simulink model "MCU_vectorControl_dsPIC33CK256MP508_LVMC"  (R2024a)
settings: Solver=FixedStepDiscrete  StartTime=0.0  StopTime=10.0  FixedStep=50e-6  RelTol=1e-3  EnableMultiTasking=on
undefined symbols (not defined in the file or in its folder): A0, A4, AN0, AN1, B0, B2, Bias1, Bias2, C12, C13, C14, C7, control, D11, D12, D13, D14, D5, D6, D7, diff, DiscIntNeverNeededParam, inverter, Max, MaxPer, model, ms, NumBits1, NumBits2, P20, P32, P55, P60, P61, P62, P69, P70, P71, P75, P76, P77, P78, Pin, pmsm, PosRange1, PosRange2, PWM1max, Resol, s, Slope1, Slope2, us
libraries: simulink x54, MCHP_Blockset x25
(part 3 of 4)

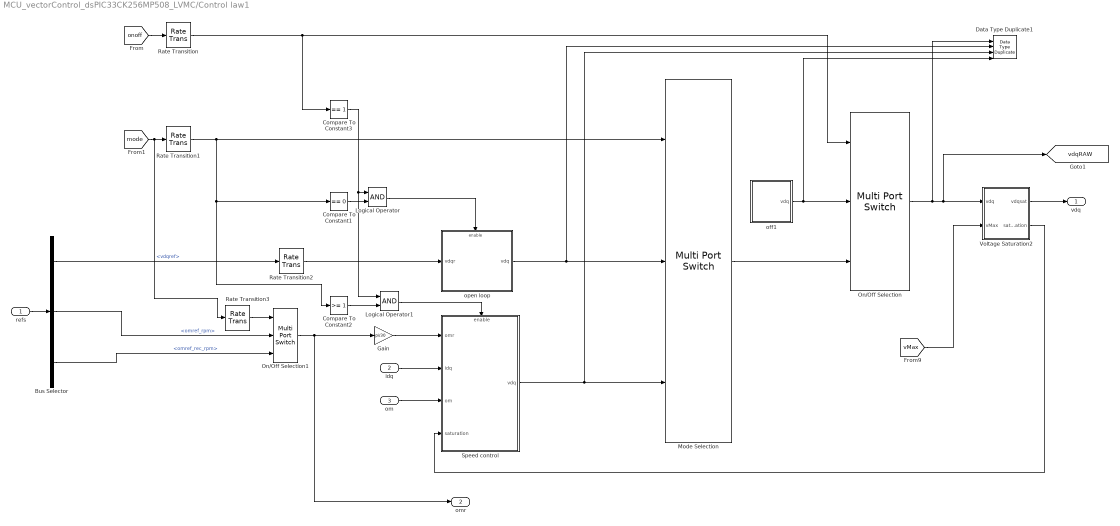
== system MCU_vectorControl_dsPIC33CK256MP508_LVMC/Control law1 ==
  refs : Inport
  idq : Inport  Port=2
  om : Inport  Port=3
  Bus Selector : BusSelector  OutputSignals=vdqref,omref.omref_rpm,omref.omref_rec_rpm
  Compare To Constant1 : simulink/Logic and Bit Operations/Compare To Constant  relop===  const=0  OutDataTypeStr=boolean
  Compare To Constant2 : simulink/Logic and Bit Operations/Compare To Constant  relop=>=  const=1  OutDataTypeStr=boolean
  Compare To Constant3 : simulink/Logic and Bit Operations/Compare To Constant  relop===  const=1  OutDataTypeStr=boolean
  Data Type Duplicate1 : DataTypeDuplicate  NumInputPorts=5
  Gain : Gain  Gain=pi/30  OutDataTypeStr=Inherit: Inherit via back propagation
  Logical Operator : Logic  AllPortsSameDT=off  OutDataTypeStr=boolean
  Logical Operator1 : Logic  AllPortsSameDT=off  OutDataTypeStr=boolean
  Mode Selection : MultiPortSwitch  DataPortOrder=Zero-based contiguous  Inputs=2  DiagnosticForDefault=None  zeroidx=on  SaturateOnIntegerOverflow=off  InputSameDT=off
  On/Off Selection : MultiPortSwitch  DataPortOrder=Zero-based contiguous  Inputs=2  DiagnosticForDefault=None  zeroidx=on  SaturateOnIntegerOverflow=off  InputSameDT=off
  On/Off Selection1 : MultiPortSwitch  DataPortOrder=Specify indices  Inputs=2  DataPortIndices={1,2}  DiagnosticForDefault=None  SaturateOnIntegerOverflow=off  InputSameDT=off
  Rate Transition{,1..3} (4 alike) : RateTransition
  Speed control : Subsystem
      settings: LibrarySourceBlock=insa_control_base/Current Control  PortSchema="{\"entries\":[{\"content\":{\"sides\":[{\"content\":{\"connectorIds\":[\"In1\",\"In2\",\"In3\",\"In4\"]},\"type\":\"ConnectorPlacement.EquallySpacedRectSide\",\"uuid\":\"e7aaa2d5-acdd-4a4d-91b1-423dc6f26e4f\"},{\"content\":{\"connectorIds\":[\"Out1\"],\"side\":\"RIGHT\"},\"type\":\"ConnectorPlacement.EquallySpacedRectSide\",\"uuid\":\"81691e4d-c138-404c-a913-2433211e99ad\"},{\"content\":{\"connectorIds\":[\"In5\"],\"side\":\"TOP\"},\"type\":\"ConnectorPlacement.EquallySpacedRectSide\",\"uuid\":\"67eaf657-96ad-4741-9677-f3dc17f9f096\"}]},\"type\":\"ConnectorPlacement.EquallySpacedConnector\",\"uuid\":\"09d68ba6-6bd5-4801-b033-56cd43b3cecf\"}],\"packageUris\":[\"http://schema.mathworks.com/mf0/Connector/R2020b\"],\"version\":\"1.0\"}"
  Voltage Saturation2 : Subsystem
  off1 : Subsystem
  open loop : Subsystem
  vdq : Outport  VectorParamsAs1DForOutWhenUnconnected=off
  omr : Outport  Port=2
  tag scope: vdqRAW=global
  wires:
  Bus Selector/1 -> Rate Transition2/1  "<vdqref>"
  [mode] -> Rate Transition1/1, Rate Transition3/1
  refs/1 -> Bus Selector/1
  Bus Selector/2 -> On/Off Selection1/2  "<omref_rpm>"
  Bus Selector/3 -> On/Off Selection1/3  "<omref_rec_rpm>"
  On/Off Selection1/1 -> omr/1, Gain/1
  Rate Transition3/1 -> On/Off Selection1/1
  [vMax] -> Voltage Saturation2/2(vMax)
  On/Off Selection/1 -> Voltage Saturation2/1(vdq), [vdqRAW], Data Type Duplicate1/2
  Speed control/1(vdq) -> Mode Selection/3, Data Type Duplicate1/4
  Voltage Saturation2/2(saturation) -> Speed control/4(saturation)
  idq/1 -> Speed control/2(idq)
  om/1 -> Speed control/3(om)
  Logical Operator1/1 -> Speed control/5(enable)
  Compare To Constant3/1 -> Logical Operator/1, Logical Operator1/1
  Compare To Constant1/1 -> Logical Operator/2
  [onoff] -> Rate Transition/1
  open loop/1(vdq) -> Mode Selection/2, Data Type Duplicate1/3
  off1/1(vdq) -> On/Off Selection/2, Data Type Duplicate1/5
  Mode Selection/1 -> On/Off Selection/3
  Logical Operator/1 -> open loop/Enable
  Compare To Constant2/1 -> Logical Operator1/2
  Voltage Saturation2/1(vdqsat) -> vdq/1
  Rate Transition/1 -> Compare To Constant3/1, On/Off Selection/1
  Rate Transition1/1 -> Mode Selection/1, Compare To Constant2/1, Compare To Constant1/1
  Rate Transition2/1 -> open loop/1(vdqr)
  Gain/1 -> Speed control/1(omr)

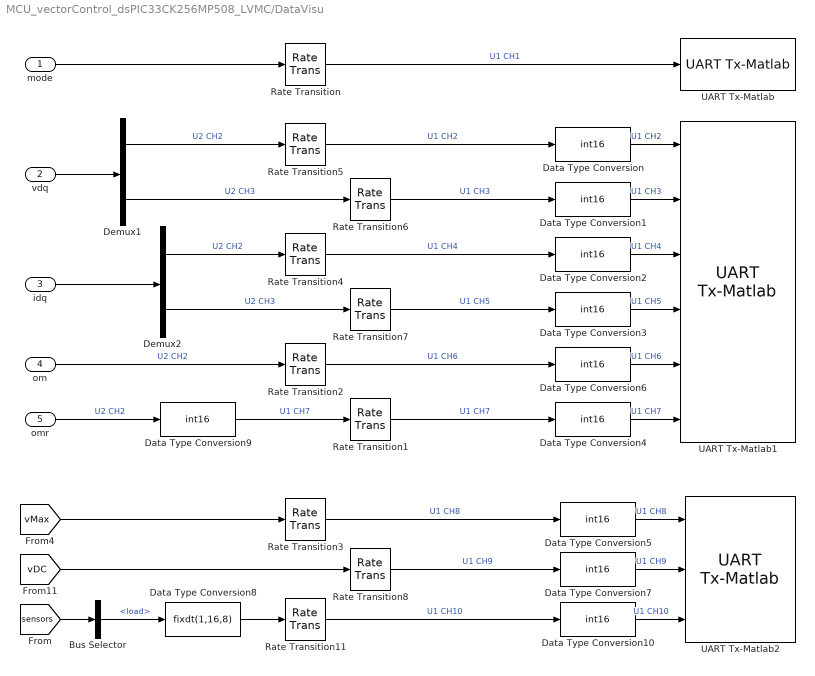
== system MCU_vectorControl_dsPIC33CK256MP508_LVMC/DataVisu ==
  mode : Inport
  vdq : Inport  Port=2
  idq : Inport  Port=3
  om : Inport  Port=4
  omr : Inport  Port=5
  Bus Selector : BusSelector  OutputSignals=MCU.load
  Data Type Conversion{,1..7,10} (9 alike) : DataTypeConversion  OutDataTypeStr=int16  ConvertRealWorld=Stored Integer (SI)  SaturateOnIntegerOverflow=off  RndMeth=Floor
  Data Type Conversion8 : DataTypeConversion  OutDataTypeStr=fixdt(1,16,8)  SaturateOnIntegerOverflow=off  RndMeth=Floor
  Data Type Conversion9 : DataTypeConversion  OutDataTypeStr=int16  SaturateOnIntegerOverflow=off  RndMeth=Floor
  Demux1 : Demux  Outputs=2
  Demux2 : Demux  Outputs=2
  Rate Transition{,1..8,11} (10 alike) : RateTransition
  UART Tx-Matlab : MCHP_Blockset/BUS UART/UART Tx-Matlab  UART_REF=1  CHANNELS=[1]  AllOrNothing=off  SampleTime=.01  MCHP_MASTERLINK=MCU_vectorControl_dsPIC33CK256MP508_LVMC/BOARD dsPIC33CK LVMC/Microchip Master  MCHP_COMPILED_INFO="CompiledSampleTime= [0.010000000000000000208   0 ];CompiledInportDataTypes=[  3 ];CompiledInportDataWidth=[1];"
      settings: SourceProductName=MPLAB Device Blocks for Simulink
  UART Tx-Matlab1 : MCHP_Blockset/BUS UART/UART Tx-Matlab  UART_REF=1  CHANNELS=[2:7]  AllOrNothing=off  SampleTime=0.001  MCHP_MASTERLINK=MCU_vectorControl_dsPIC33CK256MP508_LVMC/BOARD dsPIC33CK LVMC/Microchip Master  MCHP_COMPILED_INFO="CompiledSampleTime= [0.0010000000000000000208   0 ];CompiledInportDataTypes=[  4   4   4   4   4   4 ];CompiledInportDataWidth=[1  1  1  1  1  1];"
      settings: SourceProductName=MPLAB Device Blocks for Simulink
  UART Tx-Matlab2 : MCHP_Blockset/BUS UART/UART Tx-Matlab  UART_REF=1  CHANNELS=[8:10]  AllOrNothing=off  SampleTime=.01  MCHP_MASTERLINK=MCU_vectorControl_dsPIC33CK256MP508_LVMC/BOARD dsPIC33CK LVMC/Microchip Master  MCHP_COMPILED_INFO="CompiledSampleTime= [0.010000000000000000208   0 ];CompiledInportDataTypes=[  4   4   4 ];CompiledInportDataWidth=[1  1  1];"
      settings: SourceProductName=MPLAB Device Blocks for Simulink
  wires:
  vdq/1 -> Demux1/1
  idq/1 -> Demux2/1
  Demux2/2 -> Rate Transition7/1  "U2 CH3"
  Demux2/1 -> Rate Transition4/1  "U2 CH2"
  Rate Transition5/1 -> Data Type Conversion/1  "U1 CH2"
  Demux1/2 -> Rate Transition6/1  "U2 CH3"
  Rate Transition6/1 -> Data Type Conversion1/1  "U1 CH3"
  Rate Transition4/1 -> Data Type Conversion2/1  "U1 CH4"
  Demux1/1 -> Rate Transition5/1  "U2 CH2"
  Rate Transition7/1 -> Data Type Conversion3/1  "U1 CH5"
  Rate Transition2/1 -> Data Type Conversion6/1  "U1 CH6"
  om/1 -> Rate Transition2/1  "U2 CH2"
  Rate Transition/1 -> UART Tx-Matlab/1  "U1 CH1"
  mode/1 -> Rate Transition/1
  omr/1 -> Data Type Conversion9/1  "U2 CH2"
  Rate Transition1/1 -> Data Type Conversion4/1  "U1 CH7"
  [vDC] -> Rate Transition8/1
  [vMax] -> Rate Transition3/1
  Rate Transition3/1 -> Data Type Conversion5/1  "U1 CH8"
  Rate Transition8/1 -> Data Type Conversion7/1  "U1 CH9"
  Bus Selector/1 -> Data Type Conversion8/1  "<load>"
  Rate Transition11/1 -> Data Type Conversion10/1  "U1 CH10"
  [sensors] -> Bus Selector/1
  Data Type Conversion8/1 -> Rate Transition11/1
  Data Type Conversion3/1 -> UART Tx-Matlab1/4  "U1 CH5"
  Data Type Conversion2/1 -> UART Tx-Matlab1/3  "U1 CH4"
  Data Type Conversion6/1 -> UART Tx-Matlab1/5  "U1 CH6"
  Data Type Conversion4/1 -> UART Tx-Matlab1/6  "U1 CH7"
  Data Type Conversion/1 -> UART Tx-Matlab1/1  "U1 CH2"
  Data Type Conversion1/1 -> UART Tx-Matlab1/2  "U1 CH3"
  Data Type Conversion5/1 -> UART Tx-Matlab2/1  "U1 CH8"
  Data Type Conversion10/1 -> UART Tx-Matlab2/3  "U1 CH10"
  Data Type Conversion7/1 -> UART Tx-Matlab2/2  "U1 CH9"
  Data Type Conversion9/1 -> Rate Transition1/1  "U1 CH7"

== system MCU_vectorControl_dsPIC33CK256MP508_LVMC/Heart-beat 5Hz Blinking ==
  Delay : Delay  DelayLength=1  InitialCondition=0  SampleTime=.1
  Logical Operator : Logic  Operator=NOT  AllPortsSameDT=off  OutDataTypeStr=boolean
  Rate Transition2 : RateTransition  Deterministic=off  OutPortSampleTime=0.01
  LED1 : Outport  VectorParamsAs1DForOutWhenUnconnected=off
  wires:
  Delay/1 -> Logical Operator/1
  Logical Operator/1 -> Delay/1, Rate Transition2/1
  Rate Transition2/1 -> LED1/1

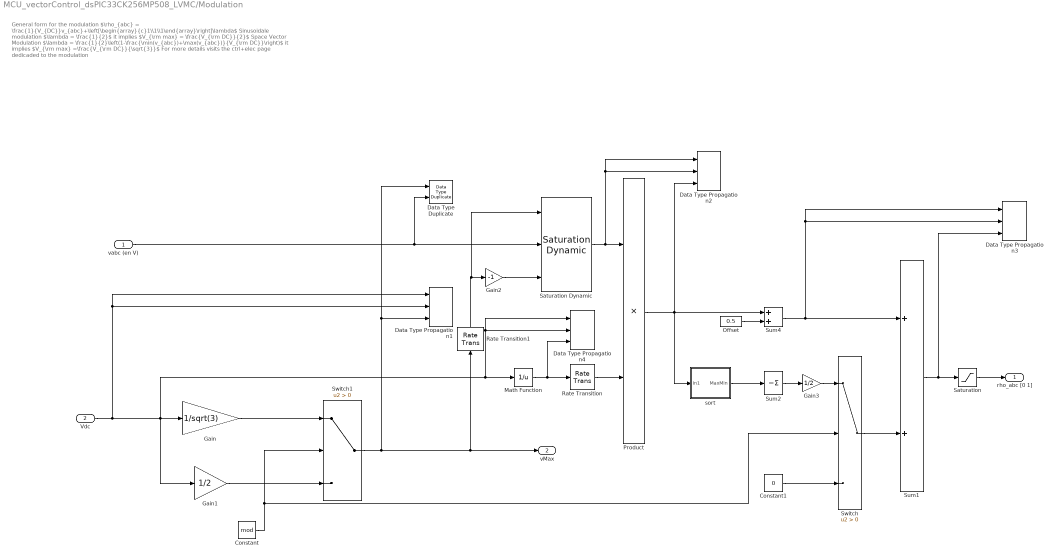
== system MCU_vectorControl_dsPIC33CK256MP508_LVMC/Modulation ==
  note: General form for the modulation
      | $\rho_{abc} = \frac{1}{V_{DC}}v_{abc}+\left[\begin{array}{c}1\\1\\1\end{array}\right]\lambda$
      | Sinusoidale modulation
      | $\lambda = \frac{1}{2}$ it implies $V_{\rm max} = \frac{V_{\rm DC}}{2}$
      | Space Vector Modulation
      | $\lambda = \frac{1}{2}\left(1-\frac{\min(v_{abc})+\max(v_{abc})}{V_{\rm DC}}\right)$ it implies $V_{\rm max} =\frac{V_{\rm DC}}{\sqrt{3}}$
      | For more details visits the ctrl+elec page dedicaded to the modulation
  "vabc (en V) " : Inport
  Vdc : Inport  Port=2
  Constant : Constant  Value=mod  OutDataTypeStr=boolean
  Constant1 : Constant  Value=0  OutDataTypeStr=Inherit: Inherit via back propagation
  Data Type Duplicate : DataTypeDuplicate
  Data Type Propagation1 : simulink/Signal Attributes/Data Type Propagation  PropDataType=fixdt(1, 16)  IfRefDouble=double  IfRefSingle=single  IsSigned=TRUE  NumBitsBase=max([NumBits1 NumBits2])  NumBitsMult=1  NumBitsAdd=0  NumBitsAllowFinal=[1:128]  PropScaling=2^-(15-ceil(log2(inverter.vDC/sqrt(3))))  ValuesUsedBestPrec=[100 -100]  SlopeBase=max([PosRange1 PosRange2])  SlopeMult=1/sqrt(3)  SlopeAdd=0  BiasBase=Bias1  BiasMult=1  BiasAdd=0
  Data Type Propagation2 : simulink/Signal Attributes/Data Type Propagation  PropDataType=fixdt(1, 16)  IfRefDouble=double  IfRefSingle=single  IsSigned=TRUE  NumBitsBase=max([NumBits1 NumBits2])  NumBitsMult=1  NumBitsAdd=0  NumBitsAllowFinal=[1:128]  PropScalingMode=Specify via dialog  PropScaling=2^-14  ValuesUsedBestPrec=[100 -100]  SlopeBase=Slope1/Slope2  SlopeMult=1  SlopeAdd=0  BiasBase=Bias1  BiasMult=1  BiasAdd=0
  Data Type Propagation3 : simulink/Signal Attributes/Data Type Propagation  PropDataType=fixdt(1, 16)  IfRefDouble=double  IfRefSingle=single  IsSigned=FALSE  NumBitsBase=max([NumBits1 NumBits2])  NumBitsMult=1  NumBitsAdd=0  NumBitsAllowFinal=[1:128]  PropScalingMode=Specify via dialog  PropScaling=2^-14  ValuesUsedBestPrec=[100 -100]  SlopeBase=Slope1/Slope2  SlopeMult=1  SlopeAdd=0  BiasBase=Bias1  BiasMult=1  BiasAdd=0
  Data Type Propagation4 : simulink/Signal Attributes/Data Type Propagation  PropDataType=fixdt(1, 16)  IfRefDouble=double  IfRefSingle=single  IsSigned=FALSE  NumBitsBase=max([NumBits1 NumBits2])  NumBitsMult=1  NumBitsAdd=0  NumBitsAllowFinal=[1:128]  PropScalingMode=Specify via dialog  PropScaling=2^-16  ValuesUsedBestPrec=[100 -100]  SlopeBase=max([PosRange1 PosRange2])  SlopeMult=1/sqrt(3)  SlopeAdd=0  BiasBase=Bias1  BiasMult=1  BiasAdd=0
  Gain : Gain  Gain=1/sqrt(3)  OutDataTypeStr=Inherit: Same as input
  Gain1 : Gain  Gain=1/2  OutDataTypeStr=Inherit: Same as input
  Gain2 : Gain  Gain=-1  ParamDataTypeStr=int16  OutDataTypeStr=Inherit: Inherit via back propagation
  Gain3 : Gain  Gain=1/2  OutDataTypeStr=Inherit: Same as input
  Math Function : Math  Operator=reciprocal  OutputSignalType=real  OutDataTypeStr=Inherit: Inherit via back propagation  SaturateOnIntegerOverflow=off
  "Offset " : Constant  Value=0.5  OutMin=[0]  OutMax=[1]  OutDataTypeStr=Inherit: Inherit via back propagation
  Product : Product  Inputs=**  OutDataTypeStr=Inherit: Inherit via back propagation  SaturateOnIntegerOverflow=on
  Rate Transition : RateTransition
  Rate Transition1 : RateTransition
  Saturation : Saturate  UpperLimit=1  LowerLimit=0
  Saturation Dynamic : simulink/Discontinuities/Saturation Dynamic  OutMin=[]  OutMax=[]  OutDataTypeStr=Inherit: Same as second input  OutDataType=fixdt(1, 16)  OutScaling=2^-10  DoSatur=off
  Sum1 : Sum  OutMin=[0]  OutMax=[1]  OutDataTypeStr=Inherit: Inherit via back propagation  InputSameDT=on  SaturateOnIntegerOverflow=on
  Sum2 : Sum  Inputs=-  OutMin=[-1]  OutMax=[1]  InputSameDT=on  SaturateOnIntegerOverflow=on  OutDataTypeStr=Inherit: Same as first input
  Sum4 : Sum  OutMin=[-1]  OutMax=[1]  InputSameDT=on  SaturateOnIntegerOverflow=on  OutDataTypeStr=Inherit: Same as first input
  Switch : Switch  Criteria=u2 > Threshold  SaturateOnIntegerOverflow=off  InputSameDT=off
  Switch1 : Switch  Criteria=u2 > Threshold  OutDataTypeStr=Inherit: Inherit via back propagation  SaturateOnIntegerOverflow=off  InputSameDT=off
  sort : Subsystem
  rho_abc [0 1] : Outport  VectorParamsAs1DForOutWhenUnconnected=off
  vMax : Outport  Port=2  VectorParamsAs1DForOutWhenUnconnected=off
  wires:
  Sum1/1 -> Saturation/1, Data Type Propagation3/3
  Vdc/1 -> Data Type Propagation1/2, Data Type Propagation1/1, Gain/1, Math Function/1, Data Type Propagation4/2, Data Type Propagation4/1, Gain1/1
  Gain3/1 -> Switch/1
  Saturation/1 -> rho_abc [0 1]/1
  Saturation Dynamic/1 -> Product/1, Data Type Propagation2/1, Data Type Propagation2/2
  Gain1/1 -> Switch1/3
  Gain/1 -> Switch1/1
  sort/1(MaxMin) -> Sum2/1
  Sum2/1 -> Gain3/1
  Sum4/1 -> Data Type Propagation3/2, Data Type Propagation3/1, Sum1/1
  Constant1/1 -> Switch/3
  Switch/1 -> Sum1/2
  "Offset "/1 -> Sum4/2
  Product/1 -> Data Type Propagation2/3, Sum4/1, sort/1(In1)
  Gain2/1 -> Saturation Dynamic/3
  Math Function/1 -> Data Type Propagation4/3, Rate Transition/1
  Switch1/1 -> Rate Transition1/1, vMax/1, Data Type Propagation1/3, Data Type Duplicate/1
  Constant/1 -> Switch1/2, Switch/2
  "vabc (en V) "/1 -> Data Type Duplicate/2, Saturation Dynamic/2
  Rate Transition/1 -> Product/2
  Rate Transition1/1 -> Saturation Dynamic/1, Gain2/1

== system MCU_vectorControl_dsPIC33CK256MP508_LVMC/Motor Choice + Gain Tunning ==

== system MCU_vectorControl_dsPIC33CK256MP508_LVMC/Park ==
  xab(c) : Inport
  P(pth) : Inport  Port=2
  Clarke : Subsystem
  Park : Subsystem
  idq : Outport
  wires:
  Park/1(xdq) -> idq/1  "idq"
  P(pth)/1 -> Park/2(P(pth))
  xab(c)/1 -> Clarke/1(xab(c))
  Clarke/1(xalphabeta) -> Park/1(xalphabeta)

== system MCU_vectorControl_dsPIC33CK256MP508_LVMC/Park inverse ==
  xdq : Inport
  P(pth) : Inport  Port=2
  Clarke Inverse : Subsystem
  Park inverse : Subsystem
  xabc : Outport
  wires:
  Park inverse/1(xalpahbeta) -> Clarke Inverse/1(xalphabeta)
  xdq/1 -> Park inverse/1(xdq)
  Clarke Inverse/1(xabc) -> xabc/1
  P(pth)/1 -> Park inverse/2(P(pth))

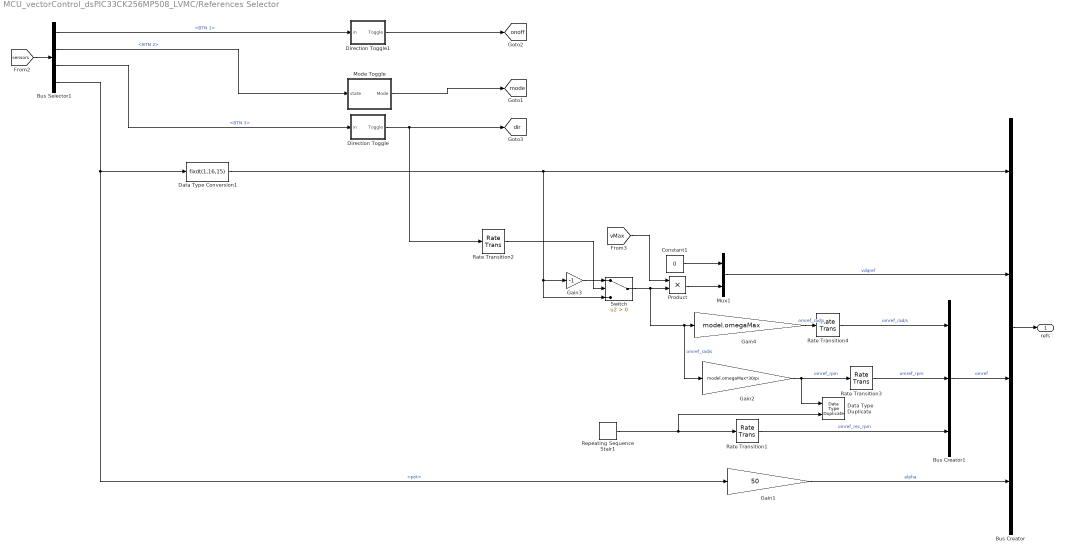
== system MCU_vectorControl_dsPIC33CK256MP508_LVMC/References Selector ==
  Bus Creator : BusCreator  Inputs=4
  Bus Creator1 : BusCreator  Inputs=3
  Bus Selector1 : BusSelector  OutputSignals=BTN.BTN 1,BTN.BTN 2,BTN.BTN 3,ADC.pot
  Constant1 : Constant  Value=0  OutDataTypeStr=Inherit: Inherit via back propagation
  Data Type Duplicate : DataTypeDuplicate
  Data Type Conversion1 : DataTypeConversion  OutDataTypeStr=fixdt(1,16,15)  SaturateOnIntegerOverflow=off  RndMeth=Floor
  Direction Toggle : Subsystem
  Direction Toggle1 : Subsystem
  Gain1 : Gain  Gain=50  OutDataTypeStr=Inherit: Inherit via back propagation
  Gain2 : Gain  Gain=model.omegaMax*30/pi  OutMax=model.omegaMax*30/pi  OutDataTypeStr=fixdt(1,16)
  Gain3 : Gain  Gain=-1  OutDataTypeStr=Inherit: Inherit via back propagation  SaturateOnIntegerOverflow=on
  Gain4 : Gain  Gain=model.omegaMax  OutMax=model.omegaMax  OutDataTypeStr=fixdt(1,16)
  Mode Toggle : Subsystem
  Mux1 : Mux  Inputs=2
  Product : Product  OutDataTypeStr=Inherit: Same as first input
  Rate Transition1 : RateTransition  OutPortSampleTime=0.001
  Rate Transition2 : RateTransition  Integrity=off  OutPortSampleTime=0.001
  Rate Transition3 : RateTransition  OutPortSampleTime=0.001
  Rate Transition4 : RateTransition  OutPortSampleTime=0.001
  Repeating Sequence Stair1 : simulink/Sources/Repeating Sequence Stair  OutValues=[1000 4000].'  tsamp=1  OutMin=[]  OutMax=[]  OutDataTypeStr=Inherit: Inherit via back propagation  OutDataType=fixdt(0,8)  ConRadixGroup=Best Precision: Vector-wise  OutScaling=2^-12
  Switch : Switch  Criteria=u2 > Threshold  OutDataTypeStr=Inherit: Inherit via back propagation  SaturateOnIntegerOverflow=off  InputSameDT=off
  refs : Outport
  tag scope: dir=global, mode=global, onoff=global
  wires:
  Rate Transition2/1 -> Switch/2
  [vMax] -> Product/1
  Gain3/1 -> Switch/1
  Mode Toggle/1(Mode) -> [mode]
  Direction Toggle1/1(Toggle) -> [onoff]
  Constant1/1 -> Mux1/1
  Mux1/1 -> Bus Creator/2  "vdqref"
  Direction Toggle/1(Toggle) -> [dir], Rate Transition2/1
  Switch/1 -> Gain2/1, Gain4/1, Product/2  "omref_rad/s"
  Bus Selector1/3 -> Direction Toggle/1(in)  "<BTN 3>"
  Bus Selector1/2 -> Mode Toggle/1(state)  "<BTN 2>"
  Bus Selector1/1 -> Direction Toggle1/1(in)  "<BTN 1>"
  [sensors] -> Bus Selector1/1
  Bus Selector1/4 -> Gain1/1, Data Type Conversion1/1  "<pot>"
  Bus Creator/1 -> refs/1
  Bus Creator1/1 -> Bus Creator/3  "omref"
  Gain2/1 -> Data Type Duplicate/1, Rate Transition3/1  "omref_rpm"
  Gain4/1 -> Rate Transition4/1  "omref_rad/s"
  Product/1 -> Mux1/2
  Gain1/1 -> Bus Creator/4  "alpha"
  Rate Transition1/1 -> Bus Creator1/3  "omref_rec_rpm"
  Repeating Sequence Stair1/1 -> Data Type Duplicate/2, Rate Transition1/1
  Rate Transition3/1 -> Bus Creator1/2  "omref_rpm"
  Rate Transition4/1 -> Bus Creator1/1  "omref_rad/s"
  Data Type Conversion1/1 -> Switch/3, Gain3/1, Bus Creator/1

== system MCU_vectorControl_dsPIC33CK256MP508_LVMC/Rot ==
  sin cos : Inport
  Demux3 : Demux  Outputs=2
  Gain : Gain  Gain=-1  OutDataTypeStr=Inherit: Same as input
  Mux1 : Mux
  Reshape : Reshape  OutputDimensionality=Customize  OutputDimensions=[2,2]
  "cos sin -sin cos " : Outport  PortDimensions=[2 2]
  wires:
  Reshape/1 -> "cos sin -sin cos "/1
  sin cos/1 -> Demux3/1
  Gain/1 -> Mux1/2
  Mux1/1 -> Reshape/1
  Demux3/1 -> Mux1/3, Gain/1
  Demux3/2 -> Mux1/4, Mux1/1

== system MCU_vectorControl_dsPIC33CK256MP508_LVMC/BOARD dsPIC33CK LVMC/ADC ==
  ADC dsPIC High Speed SAR Motor Currents : MCHP_Blockset/Analog IO/ADC dsPIC High Speed SAR  ACLKCON=Optimized for PWM resolution & ADC conversion speed  ADC_FRACT=Fractional (left aligned)  ADC_NRE=off  DMA_Size=Single trigger - (default)  ADC_Synchronisation=Triggered by custom source  ADC_Trig_TXT=PWM1 Trigger 1  ADC_TrigTimeStep=Trig model step after all sample from this block are converted  ADC_TrigInfo=0  SampleTime=50e-6  S_INPUT=[]  S_INPUT_Size=[]  S_OUTPUT="[5  5]"  S_OUTPUT_Size="[1  1]"  S_ListCustomDatatype=S.S_ListCustomDatatype={};  MCHP_USER_INTERRUPTS={ADCAN0}{ADCBUF0}{ADC Data 0 Ready}{VectorName(ADCAN0Interrupt) Priority(-1) RegisterReadClear(ADCBUF0)Config_BitSet(ADIELbits.IE0) };{ADCAN1}{ADCBUF1}{ADC Data 1 Ready}{VectorName(ADCAN1Interrupt) Priority(-1) RegisterReadClear(ADCBUF1)Config_BitSet(ADIELbits.IE1) };  MCHP_PORT={Analog Input 0}{AN0}15:2:A0;{Analog Input 1}{AN1}15:2:B2;  MCHP_MASTERLINK=MCU_vectorControl_dsPIC33CK256MP508_LVMC/BOARD dsPIC33CK LVMC/Microchip Master  MCHP_CRC=3816313  ADC_Info=Total Time = 640(ns)  ADC0_pin_TXT=AN0 / A0 / Pin[16]  ADC0_R="< 5    kOhm"  ADC0_res=12 bits  ADC0_signed=signed 16 bits  ADC0_FILTER=No Oversampling  ADC0_FILTER_nSamples=256 samples  ADC0_STRGEN=Start sampling followed by conversion  ADC0_STRGEN_on=Start sampling followed by conversion  ADC0_SSAMPEN=off  ADC0_Info=tSmp_min=260(ns) x 1 = 260(ns) ; tConv=370(ns) x 1 = 370(ns) ; TOTAL=640(ns)  ADC1_pin_TXT=AN1 / B2 / Pin[41]  ADC1_R="< 5    kOhm"  ADC1_res=12 bits  ADC1_signed=signed 16 bits  ADC1_FILTER=No Oversampling  ADC1_FILTER_nSamples=128 samples  ADC1_STRGEN=Start sampling followed by conversion  ADC1_STRGEN_on=Start sampling followed by conversion  ADC1_SSAMPEN=off  ADC1_Info=tSmp_min=260(ns) x 1 = 260(ns) ; tConv=370(ns) x 1 = 370(ns) ; TOTAL=640(ns)  ADC2_pin_TXT=Not used  ADC2_R="< 5    kOhm"  ADC2_res=12 bits  ADC2_signed=signed 16 bits  ADC2_FILTER=No Oversampling  ADC2_FILTER_nSamples=256 samples  ADC2_STRGEN=End sampling and start conversion  ADC2_STRGEN_on=Start sampling followed by conversion  ADC2_SSAMPEN=on  ADC2_Info=tSmp_min=14.706(ns) x 0 = 0(s) ; tConv=154.41(ns) x 0 = 0(s) ; TOTAL=0(s)  ADC3_pin_TXT=Not used  ADC3_R="< 10   kOhm"  ADC3_res=12 bits  ADC3_signed=signed 16 bits  ADC3_FILTER=Burst convert of n samples are Summed  ADC3_FILTER_nSamples=64 samples  ADC3_STRGEN=End sampling and start conversion  ADC3_STRGEN_on=Start sampling followed by conversion  ADC3_SSAMPEN=on  ADC3_Info=tSmp_min=14.706(ns) x 0 = 0(s) ; tConv=154.41(ns) x 0 = 0(s) ; TOTAL=0(s)  ADC4_pin_TXT=Not used  ADC4_R=< 200 Ohm  ADC4_res=12 bits  ADC4_signed=unsigned 16 bits  ADC4_FILTER=No Oversampling  ADC4_FILTER_nSamples=256 samples  ADC4_STRGEN=End sampling and start conversion  ADC4_STRGEN_on=Start sampling followed by conversion  ADC4_SSAMPEN=off  ADC4_Info=tSmp_min=14.706(ns) x 0 = 0(s) ; tConv=154.41(ns) x 0 = 0(s) ; TOTAL=0(s)  ADC5_pin_TXT=Not used  ADC5_R=< 200 Ohm  ADC5_res=12 bits  ADC5_signed=unsigned 16 bits  ADC5_FILTER=Burst convert of n samples are Summed  ADC5_FILTER_nSamples=256 samples  ADC5_STRGEN=End sampling and start conversion  ADC5_STRGEN_on=Start sampling followed by conversion  ADC5_SSAMPEN=on  ADC5_Info=tSmp_min=14.706(ns) x 0 = 0(s) ; tConv=154.41(ns) x 0 = 0(s) ; TOTAL=0(s)  ADC6_pin_TXT=Not used  ADC6_R=< 200 Ohm  ADC6_res=12 bits  ADC6_signed=unsigned 16 bits  ADC6_FILTER=Burst convert of n samples are Summed  ADC6_FILTER_nSamples=256 samples  ADC6_STRGEN=End sampling and start conversion  ADC6_STRGEN_on=Start sampling followed by conversion  ADC6_SSAMPEN=on  ADC6_Info=tSmp_min=14.706(ns) x 0 = 0(s) ; tConv=154.41(ns) x 0 = 0(s) ; TOTAL=0(s)  ADC7_R="< 5    kOhm"  ADC7_res=12 bits  ADC7_AN0=Not used  ADC7_AN1=Not used  ADC7_AN2=Not used  ADC7_AN3=Not used  ADC7_AN4=Not used  ADC7_AN5=Not used  ADC7_AN6=Not used  ADC7_AN7=Not used  ADC7_AN8=Not used  ADC7_AN9=Not used  ADC7_AN10=Not used  ADC7_AN11=Not used  ADC7_AN12=Not used  ADC7_AN13=Not used  ADC7_AN14=Not used  ADC7_AN15=Not used  ADC7_AN16=Not used  ADC7_AN17=Not used  ADC7_AN18=Not used  ADC7_AN19=Not used  ADC7_AN20=Not used  ADC7_AN21=Not used  ADC7_AN22=Not used  ADC7_AN23=Not used  ADC7_AN24=Not used  ADC7_AN25=Not used  ADC7_AN26=Not used  ADC7_AN27=Not used  ADC7_AN28=Not used  ADC7_AN29=Not used  ADC7_AN30=Not used  ADC7_AN31=Not used  IVref=Not used  IVTemp=Not used  ADC7_Info=tSmp_min=20(ns) x 0 = 0(s) ; tConv=210(ns) x 0 = 0(s) ; TOTAL=0(s)
      settings: SourceProductName=MPLAB Device Blocks for Simulink
  ADC dsPIC High Speed SAR others : MCHP_Blockset/Analog IO/ADC dsPIC High Speed SAR  ACLKCON=Not used  ADC_FRACT=Fractional (left aligned)  ADC_NRE=off  DMA_Size=Single trigger - (default)  ADC_Synchronisation=Triggered by custom source  ADC_Trig_TXT=PWM1 Trigger 1  ADC_TrigTimeStep=None (independant)  ADC_TrigInfo=0  SampleTime=50e-6  S_INPUT=[]  S_INPUT_Size=[]  S_OUTPUT="[5  5]"  S_OUTPUT_Size="[1  1]"  S_ListCustomDatatype=S.S_ListCustomDatatype={};  MCHP_USER_INTERRUPTS={ADCAN3}{ADCBUF3}{ADC Data 3 Ready}{VectorName(ADCAN3Interrupt) Priority(-1) RegisterReadClear(ADCBUF3)Config_BitSet(ADIELbits.IE3) };{ADCAN10}{ADCBUF10}{ADC Data 10 Ready}{VectorName(ADCAN10Interrupt) Priority(-1) RegisterReadClear(ADCBUF10)Config_BitSet(ADIELbits.IE10) };{ADCAN14}{ADCBUF14}{ADC Data 14 Ready}{VectorName(ADCAN14Interrupt) Priority(-1) RegisterReadClear(ADCBUF14)Config_BitSet(ADIELbits.IE14) };  MCHP_PORT={Analog Input 4}{AN4}15:2:A4;{Analog Input 11}{AN11}15:2:B9;{Analog Input 15}{AN15}15:2:C3;  MCHP_MASTERLINK=MCU_vectorControl_dsPIC33CK256MP508_LVMC/BOARD dsPIC33CK LVMC/Microchip Master  MCHP_CRC=3961681  ADC_Info=Total Time = 1.98(us)  ADC0_pin_TXT=Not used  ADC0_R="< 5    kOhm"  ADC0_res=12 bits  ADC0_signed=signed 16 bits  ADC0_FILTER=No Oversampling  ADC0_FILTER_nSamples=256 samples  ADC0_STRGEN=Start sampling followed by conversion  ADC0_STRGEN_on=Start sampling followed by conversion  ADC0_SSAMPEN=off  ADC0_Info=tSmp_min=20(ns) x 0 = 0(s) ; tConv=210(ns) x 0 = 0(s) ; TOTAL=0(s)  ADC1_pin_TXT=Not used  ADC1_R="< 5    kOhm"  ADC1_res=12 bits  ADC1_signed=signed 16 bits  ADC1_FILTER=No Oversampling  ADC1_FILTER_nSamples=128 samples  ADC1_STRGEN=Start sampling followed by conversion  ADC1_STRGEN_on=Start sampling followed by conversion  ADC1_SSAMPEN=off  ADC1_Info=tSmp_min=20(ns) x 0 = 0(s) ; tConv=210(ns) x 0 = 0(s) ; TOTAL=0(s)  ADC2_pin_TXT=Not used  ADC2_R="< 5    kOhm"  ADC2_res=12 bits  ADC2_signed=signed 16 bits  ADC2_FILTER=No Oversampling  ADC2_FILTER_nSamples=256 samples  ADC2_STRGEN=End sampling and start conversion  ADC2_STRGEN_on=Start sampling followed by conversion  ADC2_SSAMPEN=on  ADC2_Info=tSmp_min=14.706(ns) x 0 = 0(s) ; tConv=154.41(ns) x 0 = 0(s) ; TOTAL=0(s)  ADC3_pin_TXT=Not used  ADC3_R="< 10   kOhm"  ADC3_res=12 bits  ADC3_signed=signed 16 bits  ADC3_FILTER=Burst convert of n samples are Summed  ADC3_FILTER_nSamples=64 samples  ADC3_STRGEN=End sampling and start conversion  ADC3_STRGEN_on=Start sampling followed by conversion  ADC3_SSAMPEN=on  ADC3_Info=tSmp_min=14.706(ns) x 0 = 0(s) ; tConv=154.41(ns) x 0 = 0(s) ; TOTAL=0(s)  ADC4_pin_TXT=Not used  ADC4_R=< 200 Ohm  ADC4_res=12 bits  ADC4_signed=unsigned 16 bits  ADC4_FILTER=No Oversampling  ADC4_FILTER_nSamples=256 samples  ADC4_STRGEN=End sampling and start conversion  ADC4_STRGEN_on=Start sampling followed by conversion  ADC4_SSAMPEN=off  ADC4_Info=tSmp_min=14.706(ns) x 0 = 0(s) ; tConv=154.41(ns) x 0 = 0(s) ; TOTAL=0(s)  ADC5_pin_TXT=Not used  ADC5_R=< 200 Ohm  ADC5_res=12 bits  ADC5_signed=unsigned 16 bits  ADC5_FILTER=Burst convert of n samples are Summed  ADC5_FILTER_nSamples=256 samples  ADC5_STRGEN=End sampling and start conversion  ADC5_STRGEN_on=Start sampling followed by conversion  ADC5_SSAMPEN=on  ADC5_Info=tSmp_min=14.706(ns) x 0 = 0(s) ; tConv=154.41(ns) x 0 = 0(s) ; TOTAL=0(s)  ADC6_pin_TXT=Not used  ADC6_R=< 200 Ohm  ADC6_res=12 bits  ADC6_signed=unsigned 16 bits  ADC6_FILTER=Burst convert of n samples are Summed  ADC6_FILTER_nSamples=256 samples  ADC6_STRGEN=End sampling and start conversion  ADC6_STRGEN_on=Start sampling followed by conversion  ADC6_SSAMPEN=on  ADC6_Info=tSmp_min=14.706(ns) x 0 = 0(s) ; tConv=154.41(ns) x 0 = 0(s) ; TOTAL=0(s)  ADC7_R="< 5    kOhm"  ADC7_res=12 bits  ADC7_AN0=Not used  ADC7_AN1=Not used  ADC7_AN2=Not used  ADC7_AN3=Not used  ADC7_AN4=signed int16  ADC7_AN5=Not used  ADC7_AN6=Not used  ADC7_AN7=Not used  ADC7_AN8=Not used  ADC7_AN9=Not used  ADC7_AN10=Not used  ADC7_AN11=unsigned int16  ADC7_AN12=Not used  ADC7_AN13=Not used  ADC7_AN14=Not used  ADC7_AN15=unsigned int16  ADC7_AN16=Not used  ADC7_AN17=Not used  ADC7_AN18=Not used  ADC7_AN19=Not used  ADC7_AN20=Not used  ADC7_AN21=Not used  ADC7_AN22=Not used  ADC7_AN23=Not used  ADC7_AN24=Not used  ADC7_AN25=Not used  ADC7_AN26=Not used  ADC7_AN27=Not used  ADC7_AN28=Not used  ADC7_AN29=Not used  ADC7_AN30=Not used  ADC7_AN31=Not used  IVref=Not used  IVTemp=Not used  ADC7_Info=tSmp_min=280(ns) x 3 = 840(ns) ; tConv=370(ns) x 3 = 1.11(us) ; TOTAL=1.98(us)
      settings: SourceProductName=MPLAB Device Blocks for Simulink
  Ia : Outport  VectorParamsAs1DForOutWhenUnconnected=off
  Ib : Outport  Port=2  VectorParamsAs1DForOutWhenUnconnected=off
  IBus : Outport  Port=3  VectorParamsAs1DForOutWhenUnconnected=off
  pot : Outport  Port=4  VectorParamsAs1DForOutWhenUnconnected=off
  V_BUS : Outport  Port=5  VectorParamsAs1DForOutWhenUnconnected=off
  wires:
  ADC dsPIC High Speed SAR Motor Currents/2 -> Ib/1
  ADC dsPIC High Speed SAR Motor Currents/1 -> Ia/1
  ADC dsPIC High Speed SAR others/1 -> IBus/1
  ADC dsPIC High Speed SAR others/2 -> pot/1
  ADC dsPIC High Speed SAR others/3 -> V_BUS/1

== system MCU_vectorControl_dsPIC33CK256MP508_LVMC/BOARD dsPIC33CK LVMC/Center & sign reversal ==
  I_ab : Inport
  Bias Update : Inport  Port=2
  Average and Sign reverse : Sum  Inputs=+-  SaturateOnIntegerOverflow=on  OutDataTypeStr=Inherit: Same as first input
  Downsample Averaged 2000 samples remove bias : Subsystem  mask{DownSample=2000}
      mask prompts: DownSample "DownSample Factor"
  Rate Transition1 : RateTransition  Deterministic=off
  Iab : Outport
  wires:
  I_ab/1 -> Average and Sign reverse/2, Downsample Averaged 2000 samples remove bias/1(In1)
  Bias Update/1 -> Downsample Averaged 2000 samples remove bias/Enable
  Downsample Averaged 2000 samples remove bias/1(Out1) -> Rate Transition1/1
  Rate Transition1/1 -> Average and Sign reverse/1
  Average and Sign reverse/1 -> Iab/1  "I_ab_raw"

== system MCU_vectorControl_dsPIC33CK256MP508_LVMC/BOARD dsPIC33CK LVMC/Downsample Averaged x20 ==
  note: DownSample & Average by changing data scaling
  In1 : Inport
  Compare To Constant : simulink/Logic and Bit Operations/Compare To Constant  relop===  const=1  OutDataTypeStr=boolean
  Counter Limited : simulink/Sources/Counter Limited  uplimit=DownSample-1  tsamp=-1
  Data Type Duplicate : DataTypeDuplicate
  Data Type Propagation : simulink/Signal Attributes/Data Type Propagation  PropDataType=fixdt(1, 16)  IfRefDouble=double  IfRefSingle=single  IsSigned=IsSigned1 or IsSigned2  NumBitsBase=NumBits1+NumBits2  NumBitsMult=1  NumBitsAdd=0  NumBitsAllowFinal=1:128  PropScaling=2^-10  ValuesUsedBestPrec=[5 -7]  SlopeBase=Slope1  SlopeMult=1  SlopeAdd=0  BiasBase=Bias1  BiasMult=1  BiasAdd=0
  Data Type Propagation1 : simulink/Signal Attributes/Data Type Propagation  PropDataType=fixdt(1, 16)  IfRefDouble=double  IfRefSingle=single  IsSigned=IsSigned1 or IsSigned2  NumBitsBase=NumBits1+NumBits2  NumBitsMult=1  NumBitsAdd=0  NumBitsAllowFinal=1:128  PropScaling=2^-10  ValuesUsedBestPrec=[5 -7]  SlopeBase=PosRange1  SlopeMult=1  SlopeAdd=0  BiasBase=Bias1  BiasMult=1  BiasAdd=0
  Discrete-Time Integrator : DiscreteIntegrator  IntegratorMethod=Accumulation: Backward Euler  gainval=1  ExternalReset=sampled level  SampleTime=-1  OutDataTypeStr=Inherit: Inherit via back propagation  ICPrevOutput=DiscIntNeverNeededParam  ICPrevScaledInput=DiscIntNeverNeededParam
  Gain : Gain  Gain=1/DownSample  OutDataTypeStr=Inherit: Inherit via back propagation  RndMeth=Round
  Gain1 : Gain  Gain=1/DownSample  OutDataTypeStr=Inherit: Inherit via back propagation
  Rate Transition1 : RateTransition  OutPortSampleTimeOpt=Multiple of input port sample time  OutPortSampleTimeMultiple=DownSample  OutPortSampleTime=DownSample
  Rate Transition3 : RateTransition  OutPortSampleTimeOpt=Multiple of input port sample time  OutPortSampleTimeMultiple=DownSample  OutPortSampleTime=DownSample
  Terminator : Terminator
  Out1 : Outport  VectorParamsAs1DForOutWhenUnconnected=off
  wires:
  Gain1/1 -> Data Type Propagation1/3, Terminator/1
  Rate Transition1/1 -> Data Type Duplicate/1, Data Type Propagation1/1, Data Type Propagation1/2
  Gain/1 -> Out1/1, Data Type Duplicate/2
  Counter Limited/1 -> Compare To Constant/1
  Discrete-Time Integrator/1 -> Rate Transition3/1, Data Type Propagation/3
  Compare To Constant/1 -> Discrete-Time Integrator/2
  In1/1 -> Data Type Propagation/1, Data Type Propagation/2, Discrete-Time Integrator/1, Rate Transition1/1
  Rate Transition3/1 -> Gain/1, Gain1/1

== system MCU_vectorControl_dsPIC33CK256MP508_LVMC/BOARD dsPIC33CK LVMC/Downsample x20 ==
  note: DownSample & Average by changing data scaling
  In1 : Inport
  Compare To Constant : simulink/Logic and Bit Operations/Compare To Constant  relop===  const=1  OutDataTypeStr=boolean
  Counter Limited : simulink/Sources/Counter Limited  uplimit=DownSample-1  tsamp=-1
  Data Type Duplicate : DataTypeDuplicate
  Data Type Propagation : simulink/Signal Attributes/Data Type Propagation  PropDataType=fixdt(1, 16)  IfRefDouble=double  IfRefSingle=single  IsSigned=IsSigned1 or IsSigned2  NumBitsBase=NumBits1+NumBits2  NumBitsMult=1  NumBitsAdd=0  NumBitsAllowFinal=1:128  PropScaling=2^-10  ValuesUsedBestPrec=[5 -7]  SlopeBase=Slope1  SlopeMult=1  SlopeAdd=0  BiasBase=Bias1  BiasMult=1  BiasAdd=0
  Data Type Propagation1 : simulink/Signal Attributes/Data Type Propagation  PropDataType=fixdt(1, 16)  IfRefDouble=double  IfRefSingle=single  IsSigned=IsSigned1 or IsSigned2  NumBitsBase=NumBits1+NumBits2  NumBitsMult=1  NumBitsAdd=0  NumBitsAllowFinal=1:128  PropScaling=2^-10  ValuesUsedBestPrec=[5 -7]  SlopeBase=PosRange1  SlopeMult=1  SlopeAdd=0  BiasBase=Bias1  BiasMult=1  BiasAdd=0
  Discrete-Time Integrator : DiscreteIntegrator  IntegratorMethod=Accumulation: Backward Euler  gainval=1  ExternalReset=sampled level  SampleTime=-1  OutDataTypeStr=Inherit: Inherit via back propagation  ICPrevOutput=DiscIntNeverNeededParam  ICPrevScaledInput=DiscIntNeverNeededParam
  Gain : Gain  Gain=1/DownSample  OutDataTypeStr=Inherit: Inherit via back propagation  RndMeth=Round
  Gain1 : Gain  Gain=1/DownSample  OutDataTypeStr=Inherit: Inherit via back propagation
  Rate Transition1 : RateTransition  OutPortSampleTimeOpt=Multiple of input port sample time  OutPortSampleTimeMultiple=DownSample  OutPortSampleTime=DownSample
  Rate Transition3 : RateTransition  OutPortSampleTimeOpt=Multiple of input port sample time  OutPortSampleTimeMultiple=DownSample  OutPortSampleTime=DownSample
  Terminator : Terminator
  Out1 : Outport  VectorParamsAs1DForOutWhenUnconnected=off
  wires:
  Rate Transition3/1 -> Gain1/1, Gain/1
  In1/1 -> Rate Transition1/1, Discrete-Time Integrator/1, Data Type Propagation/2, Data Type Propagation/1
  Compare To Constant/1 -> Discrete-Time Integrator/2
  Discrete-Time Integrator/1 -> Data Type Propagation/3, Rate Transition3/1
  Counter Limited/1 -> Compare To Constant/1
  Gain/1 -> Data Type Duplicate/2, Out1/1
  Rate Transition1/1 -> Data Type Propagation1/2, Data Type Propagation1/1, Data Type Duplicate/1
  Gain1/1 -> Terminator/1, Data Type Propagation1/3

== system MCU_vectorControl_dsPIC33CK256MP508_LVMC/BOARD dsPIC33CK LVMC/Downsample x20 _ ==
  note: DownSample & Average by changing data scaling
  In1 : Inport
  Compare To Constant : simulink/Logic and Bit Operations/Compare To Constant  relop===  const=1  OutDataTypeStr=boolean
  Counter Limited : simulink/Sources/Counter Limited  uplimit=DownSample-1  tsamp=-1
  Data Type Duplicate : DataTypeDuplicate
  Data Type Propagation : simulink/Signal Attributes/Data Type Propagation  PropDataType=fixdt(1, 16)  IfRefDouble=double  IfRefSingle=single  IsSigned=IsSigned1 or IsSigned2  NumBitsBase=NumBits1+NumBits2  NumBitsMult=1  NumBitsAdd=0  NumBitsAllowFinal=1:128  PropScaling=2^-10  ValuesUsedBestPrec=[5 -7]  SlopeBase=Slope1  SlopeMult=1  SlopeAdd=0  BiasBase=Bias1  BiasMult=1  BiasAdd=0
  Data Type Propagation1 : simulink/Signal Attributes/Data Type Propagation  PropDataType=fixdt(1, 16)  IfRefDouble=double  IfRefSingle=single  IsSigned=IsSigned1 or IsSigned2  NumBitsBase=NumBits1+NumBits2  NumBitsMult=1  NumBitsAdd=0  NumBitsAllowFinal=1:128  PropScaling=2^-10  ValuesUsedBestPrec=[5 -7]  SlopeBase=PosRange1  SlopeMult=1  SlopeAdd=0  BiasBase=Bias1  BiasMult=1  BiasAdd=0
  Discrete-Time Integrator : DiscreteIntegrator  IntegratorMethod=Accumulation: Backward Euler  gainval=1  ExternalReset=sampled level  SampleTime=-1  OutDataTypeStr=Inherit: Inherit via back propagation  ICPrevOutput=DiscIntNeverNeededParam  ICPrevScaledInput=DiscIntNeverNeededParam
  Gain : Gain  Gain=1/DownSample  OutDataTypeStr=Inherit: Inherit via back propagation  RndMeth=Round
  Gain1 : Gain  Gain=1/DownSample  OutDataTypeStr=Inherit: Inherit via back propagation
  Rate Transition1 : RateTransition  OutPortSampleTimeOpt=Multiple of input port sample time  OutPortSampleTimeMultiple=DownSample  OutPortSampleTime=DownSample
  Rate Transition3 : RateTransition  OutPortSampleTimeOpt=Multiple of input port sample time  OutPortSampleTimeMultiple=DownSample  OutPortSampleTime=DownSample
  Terminator : Terminator
  Out1 : Outport  VectorParamsAs1DForOutWhenUnconnected=off
  wires:
  Gain1/1 -> Data Type Propagation1/3, Terminator/1
  Rate Transition1/1 -> Data Type Duplicate/1, Data Type Propagation1/1, Data Type Propagation1/2
  Gain/1 -> Out1/1, Data Type Duplicate/2
  Counter Limited/1 -> Compare To Constant/1
  Discrete-Time Integrator/1 -> Rate Transition3/1, Data Type Propagation/3
  Compare To Constant/1 -> Discrete-Time Integrator/2
  In1/1 -> Data Type Propagation/1, Data Type Propagation/2, Discrete-Time Integrator/1, Rate Transition1/1
  Rate Transition3/1 -> Gain/1, Gain1/1

== system MCU_vectorControl_dsPIC33CK256MP508_LVMC/BOARD dsPIC33CK LVMC/LVMC board webpage ==

== system MCU_vectorControl_dsPIC33CK256MP508_LVMC/BOARD dsPIC33CK LVMC/PWM Scaling ==
  vabc [0 1] : Inport
  Gain : Gain  Gain=PWM1max  OutDataTypeStr=uint16
  PWM : Outport  VectorParamsAs1DForOutWhenUnconnected=off
  wires:
  vabc [0 1]/1 -> Gain/1
  Gain/1 -> PWM/1

== system MCU_vectorControl_dsPIC33CK256MP508_LVMC/BOARD dsPIC33CK LVMC/Timing Analysis ==
  note: CPU overload is 0 if no overload took place between two MCU Overload block execution.
      | Otherwise, bits field output code for TID(s) responsible for at least one overload.
  Downsample Averaged2 : Subsystem  mask{InputSampleTime=.0005, DownSample=200}
      mask prompts: InputSampleTime "Input sample time"; DownSample "DownSample Factor"
  Gain : Gain  Gain=10e-9/.0005 * 100  OutMin=0  OutMax=100  OutDataTypeStr=fixdt(0,16)  RndMeth=Simplest  SaturateOnIntegerOverflow=on
  MCU Load : MCHP_Blockset/Profiling/MCU Load  MCULoadPin_TXT=None  MCULoadMeasure=on  TIMER_Resolution_TXT="Resol: 0.01(us)  -  Max: 0.655(ms)"  MCHP_TIMER_REQUEST={MCU_Load}{MCU_Load}21:5:0:0:[]:65536;  MCHP_TIMER_RESULT=[1 65535 ]  MCHP_MASTERLINK=MCU_vectorControl_dsPIC33CK256MP508_LVMC/BOARD dsPIC33CK LVMC/Microchip Master  MCHP_COMPILED_INFO="CompiledSampleTime= [0.00050000000000000001041   0 ];CompiledInportDataTypes=[    ];CompiledInportDataWidth=[];"  Info="Timer 1:  Resol: 10(ns)  -  Max: 655.36(us)"  SampleTime=.0005
      settings: SourceProductName=MPLAB Device Blocks for Simulink
  MCU Overload : MCHP_Blockset/Profiling/MCU Overload  MCUOverloadBlockOutput=on  MCUOverLoadPin_TXT=None  MCHP_MASTERLINK=MCU_vectorControl_dsPIC33CK256MP508_LVMC/BOARD dsPIC33CK LVMC/Microchip Master  SampleTime=-1
      settings: SourceProductName=MPLAB Device Blocks for Simulink
  Overload : Constant  Value=65535  OutDataTypeStr=Inherit: Inherit via back propagation
  Rate Transition : RateTransition  Deterministic=off  OutPortSampleTime=.0005*200
  Switch : Switch  Criteria=u2 ~= 0  SaturateOnIntegerOverflow=off  InputSameDT=off
  CPU Load : Outport  Unit=%  SampleTime=.0005*200
  CPU Overload : Outport  Port=2
  wires:
  Rate Transition/1 -> Switch/2
  MCU Overload/1 -> Rate Transition/1, CPU Overload/1
  MCU Load/1 -> Downsample Averaged2/1(In1)
  Downsample Averaged2/1(Out1) -> Switch/3
  Switch/1 -> Gain/1
  Overload/1 -> Switch/1
  Gain/1 -> CPU Load/1

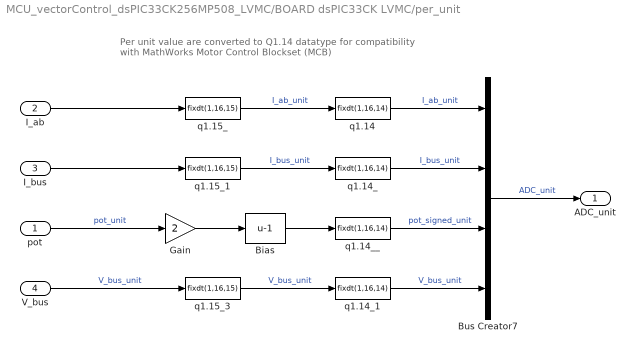
== system MCU_vectorControl_dsPIC33CK256MP508_LVMC/BOARD dsPIC33CK LVMC/per_unit ==
  note: Per unit value are converted to Q1.14 datatype
      | for compatibility with MathWorks Motor Control Blockset (MCB)
  pot : Inport
  I_ab : Inport  Port=2
  I_bus : Inport  Port=3
  V_bus : Inport  Port=4
  Bias : Bias  Bias=-1  SaturateOnIntegerOverflow=off
  Bus Creator7 : BusCreator  Inputs=4
  Gain : Gain  Gain=2  OutDataTypeStr=fixdt(1,16,15)  LockScale=on
  q1.14 : DataTypeConversion  OutDataTypeStr=fixdt(1,16,14)  SaturateOnIntegerOverflow=off  RndMeth=Floor  LockScale=on
  q1.14_ : DataTypeConversion  OutDataTypeStr=fixdt(1,16,14)  SaturateOnIntegerOverflow=off  RndMeth=Floor  LockScale=on
  q1.14_1 : DataTypeConversion  OutDataTypeStr=fixdt(1,16,14)  SaturateOnIntegerOverflow=off  RndMeth=Floor  LockScale=on
  q1.14__ : DataTypeConversion  OutDataTypeStr=fixdt(1,16,14)  SaturateOnIntegerOverflow=off  RndMeth=Floor  LockScale=on
  q1.15_ : DataTypeConversion  OutDataTypeStr=fixdt(1,16,15)  ConvertRealWorld=Stored Integer (SI)  SaturateOnIntegerOverflow=off  RndMeth=Floor  LockScale=on
  q1.15_1 : DataTypeConversion  OutDataTypeStr=fixdt(1,16,15)  ConvertRealWorld=Stored Integer (SI)  SaturateOnIntegerOverflow=off  RndMeth=Floor  LockScale=on
  q1.15_3 : DataTypeConversion  OutDataTypeStr=fixdt(1,16,15)  ConvertRealWorld=Stored Integer (SI)  SaturateOnIntegerOverflow=off  RndMeth=Floor  LockScale=on
  ADC_unit : Outport
  wires:
  I_ab/1 -> q1.15_/1
  V_bus/1 -> q1.15_3/1  "V_bus_unit"
  pot/1 -> Gain/1  "pot_unit"
  I_bus/1 -> q1.15_1/1
  q1.15_1/1 -> q1.14_/1  "I_bus_unit"
  q1.15_/1 -> q1.14/1  "I_ab_unit"
  Bus Creator7/1 -> ADC_unit/1  "ADC_unit"
  q1.15_3/1 -> q1.14_1/1  "V_bus_unit"
  q1.14/1 -> Bus Creator7/1  "I_ab_unit"
  q1.14_/1 -> Bus Creator7/2  "I_bus_unit"
  q1.14__/1 -> Bus Creator7/3  "pot_signed_unit"
  q1.14_1/1 -> Bus Creator7/4  "V_bus_unit"
  Gain/1 -> Bias/1
  Bias/1 -> q1.14__/1

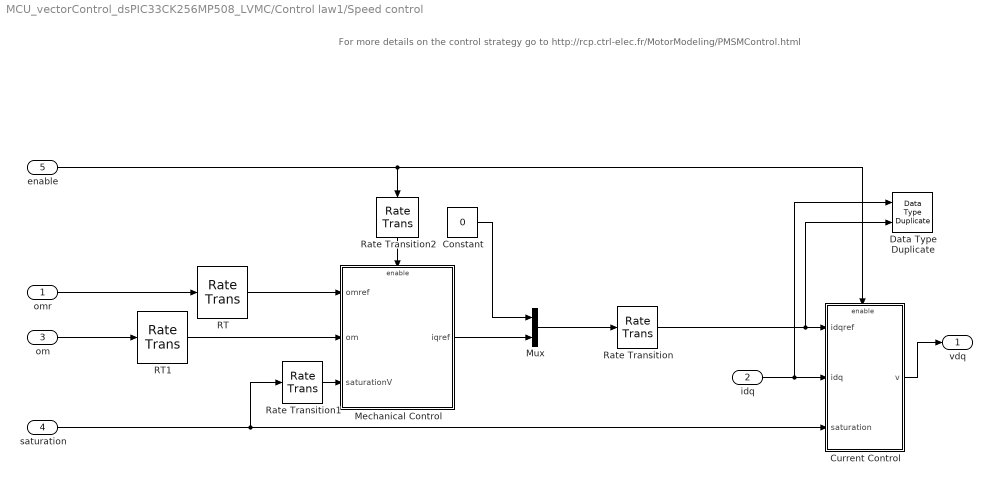
== system MCU_vectorControl_dsPIC33CK256MP508_LVMC/Control law1/Speed control ==
  note: For more details on the control strategy go to
      |
      | http://rcp.ctrl-elec.fr/MotorModeling/PMSMControl.html
  omr : Inport
  idq : Inport  Port=2
  om : Inport  Port=3
  saturation : Inport  Port=4
  enable : Inport  Port=5
  Constant : Constant  Value=0  OutDataTypeStr=Inherit: Inherit via back propagation
  Current Control : Subsystem
  Data Type Duplicate : DataTypeDuplicate
  Mechanical Control : Subsystem
  Mux : Mux  Inputs=2
  RT : RateTransition  OutPortSampleTime=0.001
  RT1 : RateTransition  OutPortSampleTime=0.001
  Rate Transition : RateTransition
  Rate Transition1 : RateTransition  OutPortSampleTime=control.tsMeca
  Rate Transition2 : RateTransition
  vdq : Outport
  wires:
  RT1/1 -> Mechanical Control/2(om)
  RT/1 -> Mechanical Control/1(omref)
  idq/1 -> Data Type Duplicate/1, Current Control/2(idq)
  Mux/1 -> Rate Transition/1
  Current Control/1(v) -> vdq/1
  saturation/1 -> Rate Transition1/1, Current Control/3(saturation)
  om/1 -> RT1/1
  Constant/1 -> Mux/1
  Mechanical Control/1(iqref) -> Mux/2
  Rate Transition/1 -> Data Type Duplicate/2, Current Control/1(idqref)
  omr/1 -> RT/1
  Rate Transition1/1 -> Mechanical Control/3(saturationV)
  enable/1 -> Current Control/Enable, Rate Transition2/1
  Rate Transition2/1 -> Mechanical Control/Enable

== system MCU_vectorControl_dsPIC33CK256MP508_LVMC/Control law1/Voltage Saturation2 ==
  vdq : Inport
  vMax : Inport  Port=2
  1/sqrt(u) : Subsystem
  Data Type Duplicate : DataTypeDuplicate  NumInputPorts=3
  Divide : Product  Inputs=***  OutDataTypeStr=Inherit: Inherit via back propagation  SaturateOnIntegerOverflow=on
  Norm L2 : Subsystem
  Rate Transition : RateTransition
  Rate Transition1 : RateTransition
  Relational Operator : RelationalOperator  Operator=>  OutDataTypeStr=boolean  RndMeth=Simplest  InputSameDT=off
  Square : Subsystem
  Sum : Sum  Inputs=|+-  OutDataTypeStr=Inherit: Inherit via back propagation  SaturateOnIntegerOverflow=on
  Switch : Switch  Criteria=u2 > Threshold  OutDataTypeStr=Inherit: Inherit via back propagation  SaturateOnIntegerOverflow=off  InputSameDT=off
  vdqsat : Outport  VectorParamsAs1DForOutWhenUnconnected=off
  saturation : Outport  Port=2  VectorParamsAs1DForOutWhenUnconnected=off
  wires:
  Divide/1 -> Switch/1
  Norm L2/1(y) -> 1/sqrt(u)/1(u), Relational Operator/1
  Switch/1 -> vdqsat/1, Data Type Duplicate/2, Sum/2
  vdq/1 -> Sum/1, Switch/3, Divide/3, Norm L2/1(In1), Data Type Duplicate/1
  Sum/1 -> saturation/1, Data Type Duplicate/3
  Relational Operator/1 -> Switch/2
  vMax/1 -> Square/1(In1), Rate Transition/1
  Square/1(y) -> Rate Transition1/1
  Rate Transition/1 -> Divide/1
  Rate Transition1/1 -> Relational Operator/2
  1/sqrt(u)/1(y) -> Divide/2

== system MCU_vectorControl_dsPIC33CK256MP508_LVMC/Control law1/off1 ==
  Mux : Mux  Inputs=2
  vd : Constant  Value=0  OutDataTypeStr=Inherit: Inherit via back propagation
  vq : Constant  Value=0  OutDataTypeStr=Inherit: Inherit via back propagation
  vdq : Outport  VectorParamsAs1DForOutWhenUnconnected=off
  wires:
  vd/1 -> Mux/1
  Mux/1 -> vdq/1
  vq/1 -> Mux/2

== system MCU_vectorControl_dsPIC33CK256MP508_LVMC/Control law1/open loop ==
  vdqr : Inport
  Enable : EnablePort
  vdq : Outport  VectorParamsAs1DForOutWhenUnconnected=off
  wires:
  vdqr/1 -> vdq/1

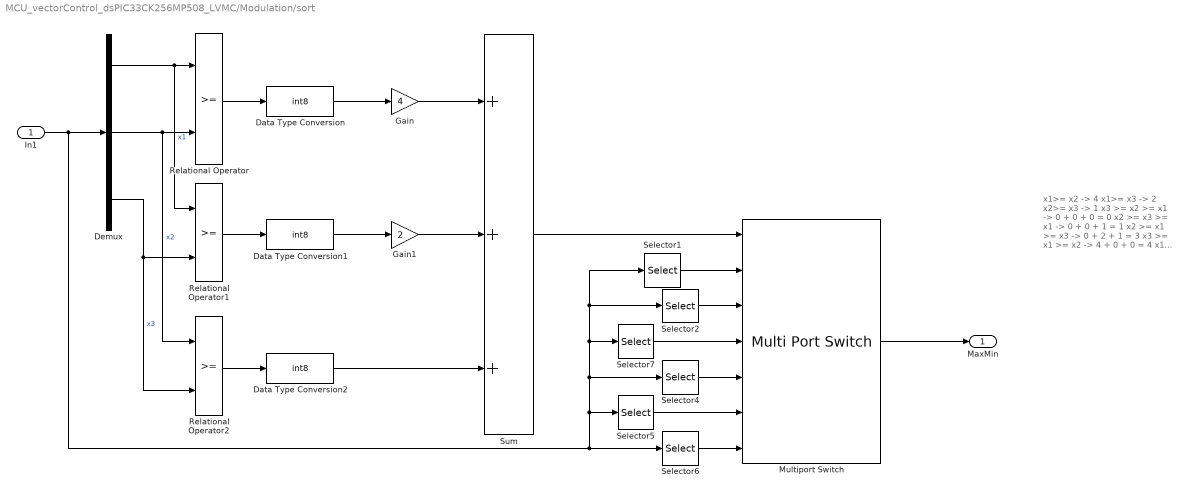
== system MCU_vectorControl_dsPIC33CK256MP508_LVMC/Modulation/sort ==
  note: x1>= x2 -> 4
      | x1>= x3 -> 2
      | x2>= x3 -> 1
      |
      | x3 >= x2 >= x1 -> 0 + 0 + 0 = 0
      | x2 >= x3 >= x1 -> 0 + 0 + 1 = 1
      | x2 >= x1 >= x3 -> 0 + 2 + 1 = 3
      | x3 >= x1 >= x2 -> 4 + 0 + 0 = 4
      | x1 >= x3 >= x2 -> 4 + 2 + 0 = 6
      | x1 >= x2 >= x3 -> 4 + 2 + 1 = 7
  In1 : Inport
  Data Type Conversion : DataTypeConversion  OutDataTypeStr=int8  SaturateOnIntegerOverflow=off  RndMeth=Floor
  Data Type Conversion1 : DataTypeConversion  OutDataTypeStr=int8  SaturateOnIntegerOverflow=off  RndMeth=Floor
  Data Type Conversion2 : DataTypeConversion  OutDataTypeStr=int8  SaturateOnIntegerOverflow=off  RndMeth=Floor
  Demux : Demux  Outputs=3
  Gain : Gain  Gain=4  OutDataTypeStr=Inherit: Same as input
  Gain1 : Gain  Gain=2  OutDataTypeStr=Inherit: Same as input
  Multiport Switch : MultiPortSwitch  DataPortOrder=Specify indices  DataPortIndices={0,1,3,4,6,7}  SaturateOnIntegerOverflow=off  InputSameDT=off
  Relational Operator : RelationalOperator  OutDataTypeStr=boolean  RndMeth=Simplest  InputSameDT=off
  Relational Operator1 : RelationalOperator  OutDataTypeStr=boolean  RndMeth=Simplest  InputSameDT=off
  Relational Operator2 : RelationalOperator  OutDataTypeStr=boolean  RndMeth=Simplest  InputSameDT=off
  Selector1 : Selector  InputPortWidth=3  IndexOptions=Index vector (dialog)  Indices=[3 1]  OutputSizes=1
  Selector2 : Selector  InputPortWidth=3  IndexOptions=Index vector (dialog)  Indices=[2 1]  OutputSizes=1
  Selector4 : Selector  InputPortWidth=3  IndexOptions=Index vector (dialog)  Indices=[3 2]  OutputSizes=1
  Selector5 : Selector  InputPortWidth=3  IndexOptions=Index vector (dialog)  Indices=[1 2]  OutputSizes=1
  Selector6 : Selector  InputPortWidth=3  IndexOptions=Index vector (dialog)  Indices=[1 3]  OutputSizes=1
  Selector7 : Selector  InputPortWidth=3  IndexOptions=Index vector (dialog)  Indices=[2 3]  OutputSizes=1
  Sum : Sum  Inputs=+++
  MaxMin : Outport
  wires:
  Demux/3 -> Relational Operator2/2, Relational Operator1/2  "x3"
  Demux/2 -> Relational Operator2/1, Relational Operator/2  "x2"
  Demux/1 -> Relational Operator1/1, Relational Operator/1  "x1"
  In1/1 -> Selector4/1, Selector7/1, Selector2/1, Selector1/1, Selector5/1, Selector6/1, Demux/1
  Relational Operator2/1 -> Data Type Conversion2/1
  Relational Operator1/1 -> Data Type Conversion1/1
  Relational Operator/1 -> Data Type Conversion/1
  Data Type Conversion/1 -> Gain/1
  Data Type Conversion1/1 -> Gain1/1
  Gain1/1 -> Sum/2
  Gain/1 -> Sum/1
  Data Type Conversion2/1 -> Sum/3
  Sum/1 -> Multiport Switch/1
  Selector1/1 -> Multiport Switch/2
  Selector6/1 -> Multiport Switch/7
  Selector5/1 -> Multiport Switch/6
  Selector4/1 -> Multiport Switch/5
  Selector7/1 -> Multiport Switch/4
  Selector2/1 -> Multiport Switch/3
  Multiport Switch/1 -> MaxMin/1

== system MCU_vectorControl_dsPIC33CK256MP508_LVMC/Park/Clarke ==
  note: Clark transform
      | $x_{\alpha\beta} = \frac{2}{3}\underbrace{\left[\begin{array}{ccc}1&-\frac{1}{2}&-\frac{1}{2}\\0&\frac{\sqrt{3}}{2}&-\frac{\sqrt{3}}{2}\end{array}\right]}_{C_{23}}x_{abc}$
      | if only 2 currents are measured since $x_a+x_b+x_c = 0$
      | $x_{abc} = \left[\begin{array}{cc}1 & 0\\0 & 1\\-1&-1\end{array}\right]x_{ab}$
      | leading to
      | $x_{\alpha\beta} = \underbrace{\left[\begin{array}{cc}1&0\\\frac{1}{\sqrt{3}}&\frac{2}{\sqrt{3}}\end{array}\right]}_{C_{22}}x_{ab}$
  xab(c) : Inport
  C1 : Gain  Gain=[1/sqrt(3) 2/sqrt(3)]  Multiplication=Matrix(K*u)  OutDataTypeStr=Inherit: Same as input
  Mux : Mux  Inputs=2
  Selector : Selector  InputPortWidth=2  IndexOptions=Index vector (dialog)  Indices=[1]  OutputSizes=1
  xalphabeta : Outport  VectorParamsAs1DForOutWhenUnconnected=off
  wires:
  xab(c)/1 -> Selector/1, C1/1
  Mux/1 -> xalphabeta/1
  Selector/1 -> Mux/1
  C1/1 -> Mux/2

== system MCU_vectorControl_dsPIC33CK256MP508_LVMC/Park/Park ==
  note: Park
      | $x_{dq} = P(\theta)^{-1}x_{\alpha\beta}\\ P(p\theta)^{-1} = \left[\begin{array}{cc}\cos(p\theta) & \sin(p\theta)\\ -\sin(p\theta) & \cos(p\theta) \end{array}\right]$
  xalphabeta : Inport  PortDimensions=2
  P(pth) : Inport  Port=2
  Data Type Duplicate2 : DataTypeDuplicate
  Park : Product  Multiplication=Matrix(*)  OutDataTypeStr=Inherit: Inherit via back propagation  RndMeth=Round
  xdq : Outport  VectorParamsAs1DForOutWhenUnconnected=off
  wires:
  Park/1 -> Data Type Duplicate2/1, xdq/1
  xalphabeta/1 -> Data Type Duplicate2/2, Park/2
  P(pth)/1 -> Park/1

== system MCU_vectorControl_dsPIC33CK256MP508_LVMC/Park inverse/Clarke Inverse ==
  note: Clarke inverse
  xalphabeta : Inport
  C23' : Gain  Gain=|  Multiplication=Matrix(K*u)  OutDataTypeStr=Inherit: Inherit via back propagation  RndMeth=Round
      | [1   -1/2        -1/2;
      |         0   sqrt(3)/2   -sqrt(3)/2]'
  xabc : Outport  VectorParamsAs1DForOutWhenUnconnected=off
  wires:
  C23'/1 -> xabc/1
  xalphabeta/1 -> C23'/1

== system MCU_vectorControl_dsPIC33CK256MP508_LVMC/Park inverse/Park inverse ==
  note: Inverse Park
      | $x_{\alpha\beta} = P(p\theta)x_{dq}\\ P(p\theta) = \left[\begin{array}{cc}\cos(p\theta) & -\sin(p\theta)\\ \sin(p\theta) & \cos(p\theta) \end{array}\right]$
  xdq : Inport
  P(pth) : Inport  Port=2
  Data Type Duplicate2 : DataTypeDuplicate
  Transpose : Math  Operator=transpose
  Transpose1 : Math  Operator=transpose
  xalpha sin(pth)1 : Product  Multiplication=Matrix(*)  OutDataTypeStr=Inherit: Inherit via back propagation  RndMeth=Round
  xalpahbeta : Outport  VectorParamsAs1DForOutWhenUnconnected=off
  wires:
  xalpha sin(pth)1/1 -> Transpose1/1, Data Type Duplicate2/1
  xdq/1 -> Transpose/1
  Transpose/1 -> xalpha sin(pth)1/1, Data Type Duplicate2/2
  Transpose1/1 -> xalpahbeta/1
  P(pth)/1 -> xalpha sin(pth)1/2
